simulink model "governor"  (R2022b)
settings: Solver=FixedStepAuto  StartTime=0.0  StopTime=10.0  FixedStep=1e-3  RelTol=1e-3
libraries: governor_lib x1
settings Model: Creator=dr_pa  LastModifiedBy=dr_pa

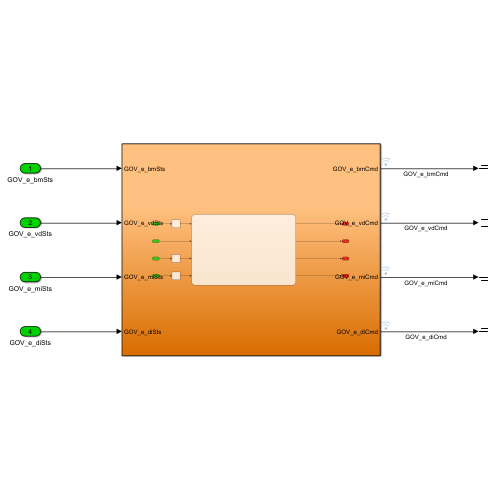
[thumbnail: Simulink's stored preview of the top-level diagram]
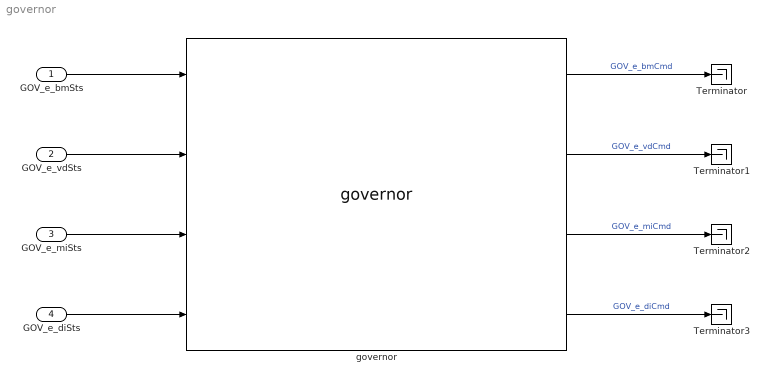
== system governor ==
  GOV_e_bmSts : Inport
  GOV_e_vdSts : Inport  Port=2
  GOV_e_miSts : Inport  Port=3
  GOV_e_diSts : Inport  Port=4
  Terminator{,1..3} (4 alike) : Terminator
  governor : governor_lib/governor  SystemSampleTime=-1  VariantActivationTime=update diagram  Latency=0  AutoFrameSizeCalculation=off
  wires:
  GOV_e_bmSts/1 -> governor/1
  GOV_e_diSts/1 -> governor/4
  GOV_e_vdSts/1 -> governor/2
  GOV_e_miSts/1 -> governor/3
  governor/1 -> Terminator/1  "GOV_e_bmCmd"
  governor/2 -> Terminator1/1  "GOV_e_vdCmd"
  governor/3 -> Terminator2/1  "GOV_e_miCmd"
  governor/4 -> Terminator3/1  "GOV_e_diCmd"
